simulink model "TF_seba"  (R2014a)
settings: Solver=ode15s  StartTime=0.0  StopTime=1  RelTol=1e-3
libraries: cstblocks x2
settings Model: Creator=lraff  LastModifiedBy=lraff

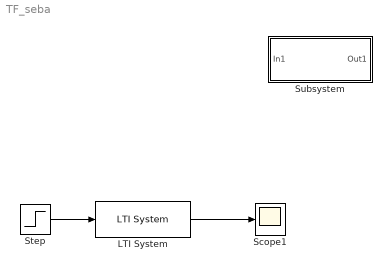
== system TF_seba ==
  LTI System : cstblocks/LTI System  sys=G  IC=[]
  Scope1 : Scope
  Step : Step  Time=0  After=440  SampleTime=0
  Subsystem : Subsystem
  wires:
  Step/1 -> LTI System/1
  LTI System/1 -> Scope1/1

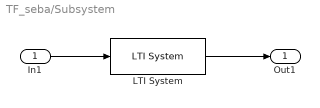
== system TF_seba/Subsystem ==
  In1 : Inport
  LTI System : cstblocks/LTI System  sys=tf(1,[1 1])  IC=[]
  Out1 : Outport
  wires:
  In1/1 -> LTI System/1
  LTI System/1 -> Out1/1
